simulink model "auv5dof2017b"  (R2018b)
settings: Solver=ode45  StartTime=0.0  StopTime=30.0  RelTol=0.05
settings Model: Creator=aditya-ubuntu  LastModifiedBy=aditya-ubuntu
settings SolverCC: MaxConsecutiveMinStep=10

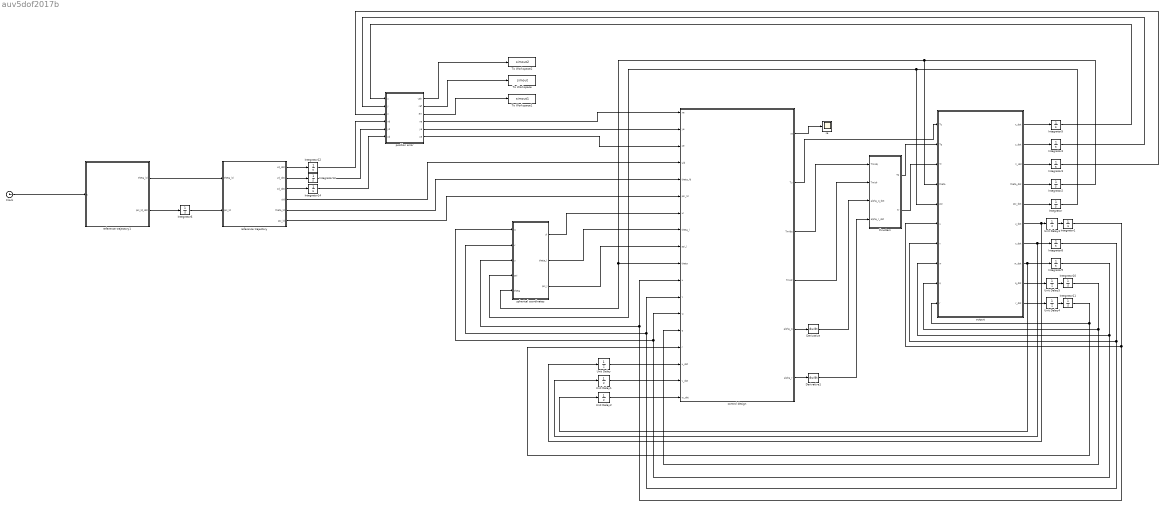
== system auv5dof2017b ==
  Clock : Clock
      settings: Decimation=100
  Derivative : Derivative
  Derivative1 : Derivative
  Integrator{,2,4,6,8..9,12} (7 alike) : Integrator
  Integrator1 : Integrator  InitialCondition=0.3  AbsoluteTolerance=0.05
  Integrator10 : Integrator  InitialCondition=0.00001
  Integrator11 : Integrator  InitialCondition=0.0000001  AbsoluteTolerance=0.05
  Integrator13 : Integrator  InitialCondition=20
  Integrator14 : Integrator  InitialCondition=5
  Integrator3 : Integrator  InitialCondition=10
  Integrator5 : Integrator  InitialCondition=10
  To Workspace : ToWorkspace  VariableName=simout  SaveFormat=Timeseries  SampleTime=-1
  To Workspace1 : ToWorkspace  VariableName=simout1  SaveFormat=Timeseries  SampleTime=-1
  To Workspace2 : ToWorkspace  VariableName=simout2  SaveFormat=Timeseries  SampleTime=-1
  Unit Delay{,1..5} (6 alike) : UnitDelay  SampleTime=-1
  control design : MATLAB Function  TreatAsAtomicUnit=on
  output : MATLAB Function  TreatAsAtomicUnit=on
  position error : MATLAB Function  TreatAsAtomicUnit=on
  re : Scope
  reference trajectory : MATLAB Function  TreatAsAtomicUnit=on
  reference trajectory1 : MATLAB Function  TreatAsAtomicUnit=on
  spherical coordinates : MATLAB Function  TreatAsAtomicUnit=on
  thrusters : MATLAB Function  TreatAsAtomicUnit=on
  wires:
  output/1(x_dot) -> Integrator5/1
  output/2(y_dot) -> Integrator4/1
  output/3(z_dot) -> Integrator3/1
  output/4(theta_dot) -> Integrator2/1
  output/5(psi_dot) -> Integrator/1
  output/6(u_dot) -> Unit Delay/1, Unit Delay3/1
  Integrator5/1 -> position error/1(x)
  Integrator4/1 -> position error/2(y)
  output/7(v_dot) -> Unit Delay1/1, Integrator8/1
  output/8(w_dot) -> Unit Delay2/1, Integrator9/1
  output/9(q_dot) -> Unit Delay5/1
  Integrator10/1 -> output/9(q), control design/14(q)
  Integrator9/1 -> output/8(w), spherical coordinates/1(w), control design/13(w)
  Integrator8/1 -> output/7(v), spherical coordinates/2(v), control design/12(v)
  Integrator1/1 -> output/6(u), spherical coordinates/3(u), control design/11(u)
  Integrator/1 -> output/5(psi), spherical coordinates/4(psi)
  Integrator2/1 -> output/4(theta), spherical coordinates/5(theta), control design/10(theta)
  Integrator11/1 -> control design/15(r), output/10(r)
  spherical coordinates/2(theta_l) -> control design/8(theta_l)
  spherical coordinates/3(psi_l) -> control design/9(psi_l)
  spherical coordinates/1(ul) -> control design/7(ul)
  reference trajectory/4(uld) -> control design/4(uld)
  Integrator3/1 -> position error/3(z)
  thrusters/1(Tq) -> output/2(Tq)
  thrusters/2(Tr) -> output/3(Tr)
  control design/4(Tmidr) -> thrusters/2(Tmidr)
  control design/3(Tmidq) -> thrusters/1(Tmidq)
  Unit Delay/1 -> control design/16(u_dot)
  Unit Delay1/1 -> control design/17(v_dot)
  Unit Delay2/1 -> control design/18(w_dot)
  Unit Delay3/1 -> Integrator1/1
  Unit Delay4/1 -> Integrator11/1
  output/10(r_dot) -> Unit Delay4/1
  control design/2(Tu) -> output/1(Tu)
  control design/1(re) -> re/1
  position error/6(ze) -> control design/3(ze)
  reference trajectory/1(xd_dot) -> Integrator12/1
  reference trajectory/2(yd_dot) -> Integrator13/1
  reference trajectory/3(zd_dot) -> Integrator14/1
  position error/5(ye) -> control design/2(ye)
  Integrator13/1 -> position error/5(yd)
  Integrator12/1 -> position error/4(xd)
  Integrator14/1 -> position error/6(zd)
  Unit Delay5/1 -> Integrator10/1
  position error/2(ref) -> To Workspace/1
  position error/3(err) -> To Workspace1/1
  position error/4(xe) -> control design/1(xe)
  position error/1(veh) -> To Workspace2/1
  control design/5(alpha_q) -> Derivative/1
  control design/6(alpha_r) -> Derivative1/1
  Derivative/1 -> thrusters/3(alpha_q_dot)
  Derivative1/1 -> thrusters/4(alpha_r_dot)
  Clock/1 -> reference trajectory1/1(t)
  reference trajectory/5(theta_ld) -> control design/5(theta_ld)
  reference trajectory/6(psi_ld) -> control design/6(psi_ld)
  reference trajectory1/1(theta_ld) -> reference trajectory/1("theta_ld ")
  reference trajectory1/2(psi_ld_dot) -> Integrator6/1
  Integrator6/1 -> reference trajectory/2("psi_ld ")

== matlab function auv5dof2017b/thrusters ==
  data: Tq output; Tr output; Tmidq input; Tmidr input; alpha_q_dot input; alpha_r_dot input
function [Tq, Tr] = fcn(Tmidq, Tmidr, alpha_q_dot, alpha_r_dot)

    m5 = 22.5;
    m6 = 15.0;
    
%     disp('Tmidq');
%     disp(Tmidq);
%     disp('Tmidr');
%     disp(Tmidr);
%     disp('alpha_q_dot');
%     disp(alpha_q_dot);
%     disp('alpha_r_dot');
%     disp(alpha_r_dot);
    
    Tq = m5*( Tmidq + alpha_q_dot);
    
    disp("Tq");
    disp(Tq);
    
    Tr = m6*( Tmidr + alpha_r_dot);
    
    disp("Tu");
    disp(Tr);
       
end

== matlab function auv5dof2017b/control design ==
  data: re output; Tu output; Tmidq output; Tmidr output; xe input; ye input; ze input; uld input; theta_ld input; psi_ld input; ul input; theta_l input; psi_l input; theta input; u input; v input; w input; q input; r input; alpha_q output; alpha_r output; u_dot input; v_dot input; w_dot input
function [re,Tu, Tmidq, Tmidr, alpha_q, alpha_r] = controlinputfn5dof(xe, ye, ze, uld, theta_ld, psi_ld, ul, theta_l, psi_l, theta, u, v, w, q, r, u_dot, v_dot, w_dot)
    
    gamma_R = 0.2;
    gamma_r = 1.2;
    gamma_q = 1.2;
    gamma_u = 1;
    gamma_psi = 0.6;
    gamma_theta = 0.6;
    
    k_psi = 0.5;
    k_theta = 0.5;
    k_R = 0.01;
    k_u = 12;
    k_r = 0.9;
    k_q = 0.9;
    
    m_u = 25.0;
    
    disp('xe');
    disp(xe);
    disp('ye');
    disp(ye);
    disp('ze');
    disp(ze);
    
    re = sqrt(xe^2 + ye^2 + ze^2);
    disp('re');
    disp(re);
    xe_dot = uld*cos(theta_ld)*cos(psi_ld) - ul*cos(theta_l)*cos(psi_l);
    ye_dot = uld*cos(theta_ld)*sin(psi_ld) - ul*cos(theta_l)*sin(psi_l);
    ze_dot = -uld*sin(theta_ld) + ul*sin(theta_l);
    
    disp('xe_dot');
    disp(xe_dot);

    disp('ye_dot');
    disp(xe_dot);

    disp('ze_dot');
    disp(xe_dot);

    theta_a = atan2(-w,sqrt(u^2+v^2));
    theta_l_D = atan2( ze, sqrt(xe^2 + ye^2) );
    theta_le = theta_l_D - theta_l;
    theta_leby2 = theta_le/2; %
    theta_leby2_inv = 2/theta_le; %
    
    theta_l_D_dot = ( ( ((xe^2 + ye^2)*ze_dot) - (ze*( xe*xe_dot + ye*ye_dot ))  ) / ( (re^2)*( sqrt(xe^2 + ye^2) ) ) ); % mine, verified
    
    alpha = theta + atan2(-w,u);
    
    B = sqrt(u^2 + w^2)/ul;
    
    b_theta = (B*cos(alpha))/sqrt(1 - ((B*sin(alpha))^2));
    
    ul_dot = (u*u_dot + v*v_dot + w*w_dot)/ul;
    
    B_dot = ( ul*(u*u_dot + w*w_dot) - (v^2+u^2)*ul_dot ) / (ul*ul*ul*B);   % mine
    
    F_theta_l = ( B_dot*sin(alpha) + (B*cos(alpha)*(u_dot*w - u*w_dot)/(u^2 + w^2))) / ( sqrt( 1 - (B*B*sin(alpha)*sin(alpha)) ) ) ;  %DOUBT in division part
    
    disp('theta_l_D_dot');
    disp(theta_l_D_dot);

    alpha_q = b_theta^(-1)*( theta_l_D_dot - F_theta_l + (gamma_theta^(-1)*( k_theta*theta_le + ( (sin(theta_leby2)*sin(theta_leby2))*theta_leby2_inv ) ) ) );
    
    disp('alpha_q');
    disp(alpha_q);
    eq = alpha_q - q;

    psi_a = atan2(v,u);
    psi_l_D = atan2(ye,xe);
    psi_le = psi_l_D - psi_l;
    
    F_psi_l = ( (u*v_dot - u_dot*v)*cos(theta) + u*v*q*sin(theta) ) / ( (u*u*cos(theta)*cos(theta)) + v^2 );
    
    psi_l_D_dot = ( xe*ye_dot - ye*xe_dot )/( xe^2 + ye^2 );
    
    alpha_r = cos(theta)*( psi_l_D_dot - F_psi_l + gamma_psi^(-1)*( k_psi*psi_le + ((sin(psi_le/2)*sin(psi_le/2))/(psi_le/2))));
    
    disp('alpha_r');
    disp(alpha_r);
    er = alpha_r - r;

    
    A = cos(theta_ld)*cos(theta_l_D)*(cos(psi_ld - psi_l_D)) + sin(theta_ld)*sin(theta_l_D);
    
    ul_D = uld*A + gamma_R^(-1)*k_R*re;
    
    A_dot = ( cos(theta_ld)*cos(theta_l_D)*sin(psi_ld - psi_l_D))*psi_l_D_dot + ( sin(theta_ld)*cos(theta_l_D) - cos(theta_ld)*sin(theta_l_D)*cos(psi_ld - psi_l_D) )*theta_l_D_dot;
    
    ule = ul_D - ul;
    
    re_dot = uld*A - ul*( cos(theta_l)*cos(theta_l_D)*cos(psi_le - 1) + cos(theta_le));
    
    ul_D_dot = uld*A_dot + gamma_R^(-1)*k_r*re_dot;
    
    Tu = m_u*sec(theta_a)*sec(psi_a)*( ul_D_dot + gamma_u^(-1)*(gamma_R*re + k_u*ule) );
    
    disp("Tu");
    disp(Tu);
    
    Tmidq = gamma_q*( k_q*eq + gamma_theta*theta_le*b_theta);
    disp("Tmidq");
    disp(Tmidq);
    
    Tmidr = gamma_r^(-1)*(k_r*er + gamma_psi*psi_le*sec(theta));
    disp("Tmidr");
    disp(Tmidr);
end

== matlab function auv5dof2017b/output ==
  settings: updateMethod=DISCRETE
  data: x_dot output; y_dot output; z_dot output; theta_dot output; psi_dot output; u_dot output; v_dot output; w_dot output; q_dot output; r_dot output; Tu input; Tq input; Tr input; theta input; psi input; u input; v input; w input; q input; r input
function [ x_dot, y_dot, z_dot, theta_dot, psi_dot, u_dot, v_dot, w_dot, q_dot, r_dot] = outputfn5dof(Tu, Tq, Tr, theta, psi, u, v, w, q, r)
    

    m = [ 25.0 17.5 30.0 1.0 22.5 15.0 ];

    onebym = [1/25.0 1/17.5 1/30.0 1.0 1/22.5 1/15.0];
    
    du = 0; %0.6848;  (1-2rand)
    dv = 0; %0.2054; % 0.3(1-2rand)
    dw = 0; %0.2054; % 0.3(1-2rand)
    dq = 0; %0.1370; % 0.2(1-2rand)
    dr = 0; %0.1370; % 0.2(1-2rand)
    
    row_g_invtri_Gml = 5.0;
   
    fu = (m(2)*v*r*onebym(1)) - (m(3)*w*q*onebym(1));
    
    fv = (-(m(1)*u*r*onebym(2)));
    
    fw = (m(1)*u*q*onebym(3));
    
    fq = ((m(3)-m(1))*u*w*onebym(5)) - ((row_g_invtri_Gml)*onebym(5)*sin(theta));
    
    fr = (m(1)-m(2))*u*v*onebym(6);
    
    x_dot = u*cos(theta)*cos(psi) - v*sin(psi) + w*sin(theta)*cos(psi);
    
    y_dot = u*cos(theta)*sin(psi) + v*cos(psi) + w*sin(theta)*sin(psi);
    
    z_dot = -u*sin(theta) + w*cos(theta);
    
    theta_dot = q;
    
    psi_dot = r*sec(theta);
    
    u_dot = fu - onebym(1)*Tu - du*u*onebym(1);
    
    v_dot = fv - dv*onebym(2)*v;
    
    w_dot = fw - dw*onebym(3)*w;
    
    q_dot = fq + onebym(5)*Tq - dq*onebym(5)*q;
    
    r_dot = fr + onebym(6)*Tr - dr*onebym(6)*r; 
    
end

== matlab function auv5dof2017b/reference trajectory ==
  data: xd_dot output; yd_dot output; zd_dot output; uld output; theta_ld output; psi_ld output; theta_ld input; psi_ld input
function [xd_dot,yd_dot,zd_dot,uld,theta_ld,psi_ld] = fcn(theta_ld,psi_ld)
    
    uld = 1.5;
    
    xd_dot = uld*cos(theta_ld)*cos(psi_ld);
    
    yd_dot = uld*cos(theta_ld)*sin(psi_ld);
    
    zd_dot = -uld*sin(theta_ld);

end

== matlab function auv5dof2017b/spherical coordinates ==
  data: w input; v input; u input; psi input; theta input; ul output; theta_l output; psi_l output
 function [ul, theta_l, psi_l] = sphericalfcn(w,v,u,psi,theta)
    
    ul = sqrt(u^2 + v^2 + w^2);
      
    %% CHECK
    

    theta_l = asin(  ( (sqrt(u^2+w^2)/ul)*(sin(theta + atan2(-w,u))) )  );
    
    psi_l = psi + atan2(u,u*cos(theta)); 

    %%DISPLAY
    disp('u');
    disp(u);
    
    disp('v');
    disp(v);
    
    disp('w');
    disp(w);
    
    disp('ul');
    disp(ul);
    disp('theta_l');
    disp(theta_l);
    disp('psi_l');
    disp(psi_l);
end

== matlab function auv5dof2017b/reference trajectory1 ==
  data: theta_ld output; psi_ld_dot output; t input
function [theta_ld,psi_ld_dot] = fcn(t)
    
    if( t<= 90)        
        theta_ld = 0;
        psi_ld_dot = 0;
    else
        theta_ld = -10;
        psi_ld_dot = 0.06;
    end

end

== matlab function auv5dof2017b/position error ==
  data: x input; y input; z input; veh output; ref output; err output; xe output; ye output; ze output; xd input; yd input; zd input

function [veh,ref,err,xe,ye,ze] = fcn(x,y,z,xd,yd,zd)
    xe = xd - x;
    
    ye = yd - y;
    
    ze = zd - z;
    
    veh = [x,y,z]';
    
    ref = [xd,yd,zd]';
    
    err = [xe,ye,ze]';
end
